simulink model "P702_NI_SoftECU"  (R2019a)
settings: Solver=ode1  StartTime=0.0  StopTime=Inf  FixedStep=0.001  RelTol=1e-3  EnableMultiTasking=on
PreLoadFcn:
  | run '.\VeriStand_BlockSet\NIVeriStandAddPaths.m'
undefined symbols (not defined in the file or in its folder): magnitude
libraries: simulink x83, simulink_extras x1
(part 68 of 76)

== system P702_NI_SoftECU/Output/Subsystem2/CAN_Signal/ECM_DIESEL PCM PCM_HEV/PowertrainData_1_0x421 ==
  AirCondFluidHi_P_Actl : Constant  Value=0
  CoolantFanStepAct : Constant  Value=0
  ECMMILRequest : Constant  Value=0
  EngIdlShutDown_D_Stat : Constant  Value=0
  EngIdlShutDwnTxt_D_Rq : Constant  Value=0
  FUEL_ALCOHOL_PERCNT : Constant  Value=0
  FohEng_D_Rq : Constant  Value=0
  OilPressureWarning : Constant  Value=0
  TrnTotLss_Tq_Est : Constant  Value=0
  TrnTotTq_Rt_Est : Constant  Value=0
  VehVLimActv_B_Actl : Constant  Value=0
  VehVLimStat_D_Actl : Constant  Value=0
  bus_creator : BusCreator  Inputs=12
  out_port : Outport
  wires:
  bus_creator/1 -> out_port/1  "Subsystem2"
  VehVLimActv_B_Actl/1 -> bus_creator/1  "VehVLimActv_B_Actl"
  VehVLimStat_D_Actl/1 -> bus_creator/2  "VehVLimStat_D_Actl"
  ECMMILRequest/1 -> bus_creator/3  "ECMMILRequest"
  FohEng_D_Rq/1 -> bus_creator/4  "FohEng_D_Rq"
  EngIdlShutDown_D_Stat/1 -> bus_creator/5  "EngIdlShutDown_D_Stat"
  CoolantFanStepAct/1 -> bus_creator/6  "CoolantFanStepAct"
  OilPressureWarning/1 -> bus_creator/7  "OilPressureWarning"
  EngIdlShutDwnTxt_D_Rq/1 -> bus_creator/8  "EngIdlShutDwnTxt_D_Rq"
  TrnTotLss_Tq_Est/1 -> bus_creator/9  "TrnTotLss_Tq_Est"
  TrnTotTq_Rt_Est/1 -> bus_creator/10  "TrnTotTq_Rt_Est"
  AirCondFluidHi_P_Actl/1 -> bus_creator/11  "AirCondFluidHi_P_Actl"
  FUEL_ALCOHOL_PERCNT/1 -> bus_creator/12  "FUEL_ALCOHOL_PERCNT"

== system P702_NI_SoftECU/Output/Subsystem2/CAN_Signal/ECM_DIESEL PCM PCM_HEV/PowertrainData_2_0x42D ==
  ApedPos_Pc_ActlDiag : Constant  Value=0
  EngAirIn_Te_Actl : Constant  Value=0
  EngClnt_Te_ActlDiag : Constant  Value=0
  EngLoad_Pc_CalcDiag : Constant  Value=0
  EngMsgTxt_D_Rq : Constant  Value=0
  GrllShtrPos_B_Falt : Constant  Value=0
  GrllShtrPos_D_Cmd : Constant  Value=0
  IsaOffst_D_Stat : Constant  Value=0
  ObdWarmUp_B_Complt : Constant  Value=0
  SlMde_D_RqDsply : Constant  Value=0
  SlMde_D_Stat : Constant  Value=0
  bus_creator : BusCreator  Inputs=11
  out_port : Outport
  wires:
  bus_creator/1 -> out_port/1  "Subsystem2"
  ObdWarmUp_B_Complt/1 -> bus_creator/1  "ObdWarmUp_B_Complt"
  EngMsgTxt_D_Rq/1 -> bus_creator/2  "EngMsgTxt_D_Rq"
  EngAirIn_Te_Actl/1 -> bus_creator/3  "EngAirIn_Te_Actl"
  ApedPos_Pc_ActlDiag/1 -> bus_creator/4  "ApedPos_Pc_ActlDiag"
  EngClnt_Te_ActlDiag/1 -> bus_creator/5  "EngClnt_Te_ActlDiag"
  EngLoad_Pc_CalcDiag/1 -> bus_creator/6  "EngLoad_Pc_CalcDiag"
  GrllShtrPos_D_Cmd/1 -> bus_creator/7  "GrllShtrPos_D_Cmd"
  GrllShtrPos_B_Falt/1 -> bus_creator/8  "GrllShtrPos_B_Falt"
  IsaOffst_D_Stat/1 -> bus_creator/9  "IsaOffst_D_Stat"
  SlMde_D_RqDsply/1 -> bus_creator/10  "SlMde_D_RqDsply"
  SlMde_D_Stat/1 -> bus_creator/11  "SlMde_D_Stat"

== system P702_NI_SoftECU/Output/Subsystem2/CAN_Signal/ECM_DIESEL PCM PCM_HEV/PowertrainData_3_0x43E ==
  BattULoChrg_U_Cmd : Constant  Value=0
  ElLoadCtl_D_Rq : Constant  Value=0
  EngMnfld_P_Actl : Constant  Value=0
  FuelPumpPwr_B_Rq : Constant  Value=0
  bus_creator : BusCreator  Inputs=4
  out_port : Outport
  wires:
  bus_creator/1 -> out_port/1  "Subsystem2"
  BattULoChrg_U_Cmd/1 -> bus_creator/1  "BattULoChrg_U_Cmd"
  ElLoadCtl_D_Rq/1 -> bus_creator/2  "ElLoadCtl_D_Rq"
  FuelPumpPwr_B_Rq/1 -> bus_creator/3  "FuelPumpPwr_B_Rq"
  EngMnfld_P_Actl/1 -> bus_creator/4  "EngMnfld_P_Actl"

== system P702_NI_SoftECU/Output/Subsystem2/CAN_Signal/ECM_DIESEL PCM PCM_HEV/PowertrainData_6_0x205 ==
  BrkTot_Tq_RqFapLc : Constant  Value=0
  FapLc_B_Err : Constant  Value=0
  TrnAin_Pc_RqDrv : Constant  Value=0
  bus_creator : BusCreator  Inputs=3
  out_port : Outport
  wires:
  bus_creator/1 -> out_port/1  "Subsystem2"
  BrkTot_Tq_RqFapLc/1 -> bus_creator/1  "BrkTot_Tq_RqFapLc"
  FapLc_B_Err/1 -> bus_creator/2  "FapLc_B_Err"
  TrnAin_Pc_RqDrv/1 -> bus_creator/3  "TrnAin_Pc_RqDrv"

== system P702_NI_SoftECU/Output/Subsystem2/CAN_Signal/ECM_DIESEL PCM PCM_HEV/PowertrainData_7_0x41F ==
  EcoCochA_Pc_Dsply : Constant  Value=0
  EcoCochCrus_Pc_Dsply : Constant  Value=0
  EcoCochDecel_Pc_Dsply : Constant  Value=0
  EcoCochIdlFuel_Pc_Dsply : Constant  Value=0
  EcoCochInstNeg_B_Dsply : Constant  Value=0
  EcoCochInst_Pc_Dsply : Constant  Value=0
  EcoCochShif_Pc_Dsply : Constant  Value=0
  bus_creator : BusCreator  Inputs=7
  out_port : Outport
  wires:
  bus_creator/1 -> out_port/1  "Subsystem2"
  EcoCochA_Pc_Dsply/1 -> bus_creator/1  "EcoCochA_Pc_Dsply"
  EcoCochCrus_Pc_Dsply/1 -> bus_creator/2  "EcoCochCrus_Pc_Dsply"
  EcoCochDecel_Pc_Dsply/1 -> bus_creator/3  "EcoCochDecel_Pc_Dsply"
  EcoCochIdlFuel_Pc_Dsply/1 -> bus_creator/4  "EcoCochIdlFuel_Pc_Dsply"
  EcoCochShif_Pc_Dsply/1 -> bus_creator/5  "EcoCochShif_Pc_Dsply"
  EcoCochInst_Pc_Dsply/1 -> bus_creator/6  "EcoCochInst_Pc_Dsply"
  EcoCochInstNeg_B_Dsply/1 -> bus_creator/7  "EcoCochInstNeg_B_Dsply"

== system P702_NI_SoftECU/Output/Subsystem2/CAN_Signal/ECM_DIESEL PCM PCM_HEV/PowertrainData_9_0x44C ==
  AutoTowActv_B_Stat : Constant  Value=0
  AutoTowAllw_D_StatMnu : Constant  Value=0
  GrossTrainWeight_M_Est : Constant  Value=0
  TrailCtlPt_B_Falt : Constant  Value=0
  Veh_V_DsplyTrailCtlSet : Constant  Value=0
  WakeAlarm1_B_Typ : Constant  Value=0
  WakeAlarm1_T_Rq : Constant  Value=0
  bus_creator : BusCreator  Inputs=7
  out_port : Outport
  wires:
  bus_creator/1 -> out_port/1  "Subsystem2"
  GrossTrainWeight_M_Est/1 -> bus_creator/1  "GrossTrainWeight_M_Est"
  AutoTowAllw_D_StatMnu/1 -> bus_creator/2  "AutoTowAllw_D_StatMnu"
  AutoTowActv_B_Stat/1 -> bus_creator/3  "AutoTowActv_B_Stat"
  TrailCtlPt_B_Falt/1 -> bus_creator/4  "TrailCtlPt_B_Falt"
  Veh_V_DsplyTrailCtlSet/1 -> bus_creator/5  "Veh_V_DsplyTrailCtlSet"
  WakeAlarm1_T_Rq/1 -> bus_creator/6  "WakeAlarm1_T_Rq"
  WakeAlarm1_B_Typ/1 -> bus_creator/7  "WakeAlarm1_B_Typ"

== system P702_NI_SoftECU/Output/Subsystem2/CAN_Signal/ECM_DIESEL PCM PCM_HEV/Powertrain_Data_4_0x424 ==
  BpedDrvMsgTxt_B_Dsply : Constant  Value=0
  FuelLvlWarn_D_ActlEng : Constant  Value=0
  FuelLvl_Pc_DsplyEng : Constant  Value=0
  FuelRange_L_DsplyEng : Constant  Value=0
  RearDiffOilTeWarn_B_Rq : Constant  Value=0
  RearDiffOil_Te_Actl : Constant  Value=0
  SelDrvMdePt_D_Stat : Constant  Value=0
  bus_creator : BusCreator  Inputs=7
  out_port : Outport
  wires:
  bus_creator/1 -> out_port/1  "Subsystem2"
  BpedDrvMsgTxt_B_Dsply/1 -> bus_creator/1  "BpedDrvMsgTxt_B_Dsply"
  RearDiffOil_Te_Actl/1 -> bus_creator/2  "RearDiffOil_Te_Actl"
  RearDiffOilTeWarn_B_Rq/1 -> bus_creator/3  "RearDiffOilTeWarn_B_Rq"
  FuelLvlWarn_D_ActlEng/1 -> bus_creator/4  "FuelLvlWarn_D_ActlEng"
  SelDrvMdePt_D_Stat/1 -> bus_creator/5  "SelDrvMdePt_D_Stat"
  FuelRange_L_DsplyEng/1 -> bus_creator/6  "FuelRange_L_DsplyEng"
  FuelLvl_Pc_DsplyEng/1 -> bus_creator/7  "FuelLvl_Pc_DsplyEng"

== system P702_NI_SoftECU/Output/Subsystem2/CAN_Signal/ECM_DIESEL PCM PCM_HEV/Powertrain_Data_5_0x43F ==
  FapLcActv_B_Stat : Constant  Value=0
  FapLcInhbt_B_Rq : Constant  Value=0
  FapLcMaxGrdAbrt_B_Stat : Constant  Value=0
  FapLcMaxGrdInhbt_B_Stat : Constant  Value=0
  FapLcObstcl_B_Stat : Constant  Value=0
  FapLcPrchgBrk_B_Rq : Constant  Value=0
  FapLcStopHold_B_Rq : Constant  Value=0
  bus_creator : BusCreator  Inputs=7
  out_port : Outport
  wires:
  bus_creator/1 -> out_port/1  "Subsystem2"
  FapLcActv_B_Stat/1 -> bus_creator/1  "FapLcActv_B_Stat"
  FapLcMaxGrdAbrt_B_Stat/1 -> bus_creator/2  "FapLcMaxGrdAbrt_B_Stat"
  FapLcMaxGrdInhbt_B_Stat/1 -> bus_creator/3  "FapLcMaxGrdInhbt_B_Stat"
  FapLcObstcl_B_Stat/1 -> bus_creator/4  "FapLcObstcl_B_Stat"
  FapLcPrchgBrk_B_Rq/1 -> bus_creator/5  "FapLcPrchgBrk_B_Rq"
  FapLcStopHold_B_Rq/1 -> bus_creator/6  "FapLcStopHold_B_Rq"
  FapLcInhbt_B_Rq/1 -> bus_creator/7  "FapLcInhbt_B_Rq"

== system P702_NI_SoftECU/Output/Subsystem2/CAN_Signal/ECM_DIESEL PCM PCM_HEV/Stop_Start_0x166 ==
  AutoStopPtDelta_I_Est : Constant  Value=0
  HiElPwInhbt_B_Stat : Constant  Value=0
  OdoTripVerify_L_Actl : Constant  Value=0
  StopStrtDrvMde_D_Indic : Constant  Value=0
  StopStrtIODTxt_D_Rq : Constant  Value=0
  StopStrtMsgTxt_D_Rq : Constant  Value=0
  StopStrtStdby_D_Indic : Constant  Value=0
  bus_creator : BusCreator  Inputs=7
  out_port : Outport
  wires:
  bus_creator/1 -> out_port/1  "Subsystem2"
  AutoStopPtDelta_I_Est/1 -> bus_creator/1  "AutoStopPtDelta_I_Est"
  HiElPwInhbt_B_Stat/1 -> bus_creator/2  "HiElPwInhbt_B_Stat"
  StopStrtDrvMde_D_Indic/1 -> bus_creator/3  "StopStrtDrvMde_D_Indic"
  StopStrtMsgTxt_D_Rq/1 -> bus_creator/4  "StopStrtMsgTxt_D_Rq"
  OdoTripVerify_L_Actl/1 -> bus_creator/5  "OdoTripVerify_L_Actl"
  StopStrtStdby_D_Indic/1 -> bus_creator/6  "StopStrtStdby_D_Indic"
  StopStrtIODTxt_D_Rq/1 -> bus_creator/7  "StopStrtIODTxt_D_Rq"

== system P702_NI_SoftECU/Output/Subsystem2/CAN_Signal/ECM_DIESEL PCM PCM_HEV/TesterPhysicalResPCM_0x7E8 ==
  TesterPhysicalResPCM : Constant  Value=0
  bus_creator : BusCreator  Inputs=1
  out_port : Outport
  wires:
  bus_creator/1 -> out_port/1  "Subsystem2"
  TesterPhysicalResPCM/1 -> bus_creator/1  "TesterPhysicalResPCM"

== system P702_NI_SoftECU/Output/Subsystem2/CAN_Signal/ECM_DIESEL PCM PCM_HEV/TorqueDataEngFlags_0x200 ==
  PrplWhlTotTqRq_No_Cnt : Constant  Value=0
  PrplWhlTotTqRq_No_Cs : Constant  Value=0
  PrplWhlTot_Tq_LimMn : Constant  Value=0
  PrplWhlTot_Tq_Rq : Constant  Value=0
  PtDrvMde_D_Stat : Constant  Value=0
  bus_creator : BusCreator  Inputs=5
  out_port : Outport
  wires:
  bus_creator/1 -> out_port/1  "Subsystem2"
  PrplWhlTot_Tq_LimMn/1 -> bus_creator/1  "PrplWhlTot_Tq_LimMn"
  PrplWhlTot_Tq_Rq/1 -> bus_creator/2  "PrplWhlTot_Tq_Rq"
  PtDrvMde_D_Stat/1 -> bus_creator/3  "PtDrvMde_D_Stat"
  PrplWhlTotTqRq_No_Cnt/1 -> bus_creator/4  "PrplWhlTotTqRq_No_Cnt"
  PrplWhlTotTqRq_No_Cs/1 -> bus_creator/5  "PrplWhlTotTqRq_No_Cs"

== system P702_NI_SoftECU/Output/Subsystem2/CAN_Signal/ECM_DIESEL PCM PCM_HEV/TransGearData ==
  GboxOil_Te_Actl : Constant  Value=0
  GearLvrPos_D_Actl : Constant  Value=0
  SelDrvMdeSwtch_D_Stat3 : Constant  Value=0
  TrnShifActv_B_Actl : Constant  Value=0
  TrnSrvcRqd_B_Rq : Constant  Value=0
  bus_creator : BusCreator  Inputs=5
  out_port : Outport
  wires:
  bus_creator/1 -> out_port/1  "Subsystem2"
  GboxOil_Te_Actl/1 -> bus_creator/1  "GboxOil_Te_Actl"
  GearLvrPos_D_Actl/1 -> bus_creator/2  "GearLvrPos_D_Actl"
  SelDrvMdeSwtch_D_Stat3/1 -> bus_creator/3  "SelDrvMdeSwtch_D_Stat3"
  TrnShifActv_B_Actl/1 -> bus_creator/4  "TrnShifActv_B_Actl"
  TrnSrvcRqd_B_Rq/1 -> bus_creator/5  "TrnSrvcRqd_B_Rq"

== system P702_NI_SoftECU/Output/Subsystem2/CAN_Signal/ECM_DIESEL PCM PCM_HEV/VehicleOperatingModes_0x167 ==
  ElPw_D_Stat : Constant  Value=0
  ElPw_D_StatStrtStop : Constant  Value=0
  Eng_D_Stat : Constant  Value=0
  PlgActvArb_B_Actl : Constant  Value=0
  PrplWhlRgenMn_Tq_Actl : Constant  Value=0
  PrplWhlTot2_Tq_Actl : Constant  Value=0
  PwPckTq_D_Stat : Constant  Value=0
  TrnAinTq_D_Qf : Constant  Value=0
  TrnAin_Tq_Actl : Constant  Value=0
  bus_creator : BusCreator  Inputs=9
  out_port : Outport
  wires:
  bus_creator/1 -> out_port/1  "Subsystem2"
  Eng_D_Stat/1 -> bus_creator/1  "Eng_D_Stat"
  PwPckTq_D_Stat/1 -> bus_creator/2  "PwPckTq_D_Stat"
  ElPw_D_Stat/1 -> bus_creator/3  "ElPw_D_Stat"
  PlgActvArb_B_Actl/1 -> bus_creator/4  "PlgActvArb_B_Actl"
  PrplWhlTot2_Tq_Actl/1 -> bus_creator/5  "PrplWhlTot2_Tq_Actl"
  ElPw_D_StatStrtStop/1 -> bus_creator/6  "ElPw_D_StatStrtStop"
  PrplWhlRgenMn_Tq_Actl/1 -> bus_creator/7  "PrplWhlRgenMn_Tq_Actl"
  TrnAinTq_D_Qf/1 -> bus_creator/8  "TrnAinTq_D_Qf"
  TrnAin_Tq_Actl/1 -> bus_creator/9  "TrnAin_Tq_Actl"

== system P702_NI_SoftECU/Output/Subsystem2/CAN_Signal/GWM/GSM ==
  in : Inport
  Gear_Shift_by_Wire_2_FD1_168 : Subsystem
  Gear_Shift_by_Wire_FD1_5A : Subsystem
  bus_creator : BusCreator  Inputs=2
  bus_selector : BusSelector  OutputSignals=Gear_Shift_by_Wire_2_FD1_168,Gear_Shift_by_Wire_FD1_5A
  out_port : Outport
  wires:
  bus_creator/1 -> out_port/1  "Subsystem2"
  Gear_Shift_by_Wire_2_FD1_168/1(out_port) -> bus_creator/1  "Gear_Shift_by_Wire_2_FD1_168"
  Gear_Shift_by_Wire_FD1_5A/1(out_port) -> bus_creator/2  "Gear_Shift_by_Wire_FD1_5A"
  in/1 -> bus_selector/1

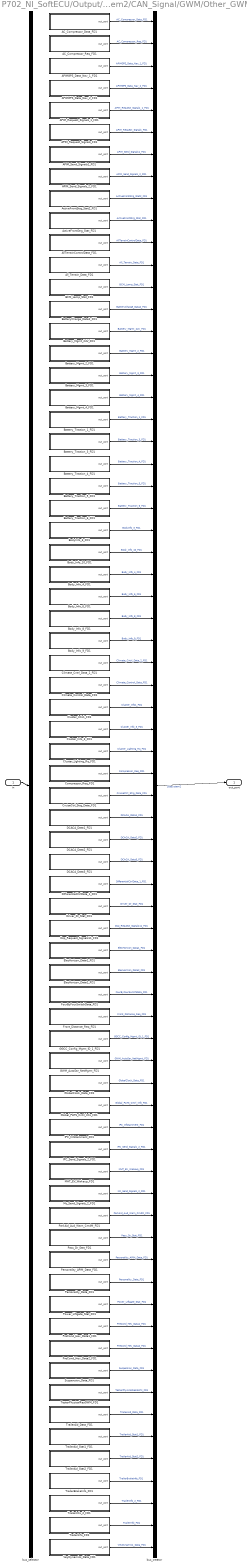
== system P702_NI_SoftECU/Output/Subsystem2/CAN_Signal/GWM/Other_GWMTx ==
  in : Inport
  AC_Compressor_Data_FD1 : Subsystem
  AC_Compressor_Req_FD1 : Subsystem
  APIMGPS_Data_Nav_1_FD1 : Subsystem
  APIMGPS_Data_Nav_2_FD1 : Subsystem
  APIM_Request_Signals_1_FD1 : Subsystem
  APIM_Request_Signals_FD1 : Subsystem
  APIM_Send_Signals1_FD1 : Subsystem
  APIM_Send_Signals_2_FD1 : Subsystem
  ActiveFrontStrg_Stat2_FD1 : Subsystem
  ActiveFrontStrg_Stat_FD1 : Subsystem
  AllTerrainControlData_FD1 : Subsystem
  All_Terrain_Data_FD1 : Subsystem
  BCM_Lamp_Stat_FD1 : Subsystem
  BatteryCharge_Data2_FD1 : Subsystem
  Battery_Mgmt_24V_FD1 : Subsystem
  Battery_Mgmt_2_FD1 : Subsystem
  Battery_Mgmt_3_FD1 : Subsystem
  Battery_Mgmt_4_FD1 : Subsystem
  Battery_Traction_1_FD1 : Subsystem
  Battery_Traction_3_FD1 : Subsystem
  Battery_Traction_4_FD1 : Subsystem
  Battery_Traction_5_FD1 : Subsystem
  Battery_Traction_6_FD1 : Subsystem
  BodyInfo_3_FD1 : Subsystem
  Body_Info_10_FD1 : Subsystem
  Body_Info_4_FD1 : Subsystem
  Body_Info_6_FD1 : Subsystem
  Body_Info_8_FD1 : Subsystem
  Body_Info_9_FD1 : Subsystem
  Climate_Cntrl_Data_2_FD1 : Subsystem
  Climate_Control_Data_FD1 : Subsystem
  Cluster_Info1_FD1 : Subsystem
  Cluster_Info_3_FD1 : Subsystem
  Cluster_Lighting_Rq_FD1 : Subsystem
  Compressor_Req_FD1 : Subsystem
  CruiseCtrl_Strg_Data_FD1 : Subsystem
  DCACA_Data1_FD1 : Subsystem
  DCACA_Data2_FD1 : Subsystem
  DCACA_Data3_FD1 : Subsystem
  DifferentialCtrlData_1_FD1 : Subsystem
  Driver_Dr_Stat_FD1 : Subsystem
  Dsp_Request_Signals11_FD1 : Subsystem
  ElecHorizon_Data1_FD1 : Subsystem
  ElecHorizon_Data2_FD1 : Subsystem
  FourByFourSwitchData_FD1 : Subsystem
  Front_Distance_Req_FD1 : Subsystem
  GGCC_Config_Mgmt_ID_1_FD1 : Subsystem
  GWM_AutoSar_NetMgmt_FD1 : Subsystem
  GlobalClock_Data_FD1 : Subsystem
  Global_PATS_Cntrl_Info_FD1 : Subsystem
  IPC_Infotainment_FD1 : Subsystem
  IPC_Send_Signals_2_FD1 : Subsystem
  MHT_EV_Wakeup_FD1 : Subsystem
  Mc_Send_Signals_2_FD1 : Subsystem
  ParkAid_Aud_Warn_CmdM_FD1 : Subsystem
  Pass_Dr_Stat_FD1 : Subsystem
  Personality_APIM_Data_FD1 : Subsystem
  Personality_Data_FD1 : Subsystem
  Power_Liftgate_Stat_FD1 : Subsystem
  PreCond_Hev_Data1_FD1 : Subsystem
  PreCond_Hev_Data2_FD1 : Subsystem
  Suspension_Data_FD1 : Subsystem
  TesterPhysicalResGWM_FD1 : Subsystem
  TrailerAid_Data_FD1 : Subsystem
  TrailerAid_Stat1_FD1 : Subsystem
  TrailerAid_Stat2_FD1 : Subsystem
  TrailerBrakeInfo_FD1 : Subsystem
  TrailerInfo_2_FD1 : Subsystem
  TrailerInfo_FD1 : Subsystem
  VeyDynamics_Data_FD1 : Subsystem
  bus_creator : BusCreator  Inputs=70
  bus_selector : BusSelector  OutputSignals=AC_Compressor_Data_FD1,AC_Compressor_Req_FD1,APIMGPS_Data_Nav_1_FD1,APIMGPS_Data_Nav_2_FD1,APIM_Request_Signals_1_FD1,APIM_Request_Signals_FD1,APIM_Send_Signals1_FD1,APIM_Send_Signals_2_FD1,ActiveFrontStrg_Stat2_FD1,ActiveFrontStrg_Stat_FD1,AllTerrainControlData_FD1,All_Terrain_Data_FD1,BCM_Lamp_Stat_FD1,BatteryCharge_Data2_FD1,Battery_Mgmt_24V_FD1,Battery_Mgmt_2_FD1,Battery_Mgmt_3_FD1,Battery_Mgmt_4_FD1,Battery_Traction_1_FD1,Battery_Traction_3_FD1,Battery_Traction_4_FD1,Battery_Traction_5_FD1,Battery_Traction_6_FD1,BodyInfo_3_FD1,Body_Info_10_FD1,Body_Info_4_FD1,Body_Info_6_FD1,Body_Info_8_FD1,Body_Info_9_FD1,Climate_Cntrl_Data_2_FD1,Climate_Control_Data_FD1,Cluster_Info1_FD1,Cluster_Info_3_FD1,Cluster_Lighting_Rq_FD1,Compressor_Req_FD1,CruiseCtrl_Strg_Data_FD1,DCACA_Data1_FD1,DCACA_Data2_FD1,DCACA_Data3_FD1,DifferentialCtrlData_1_FD1,Driver_Dr_Stat_FD1,Dsp_Request_Signals11_FD1,ElecHorizon_Data1_FD1,ElecHorizon_Data2_FD1,FourByFourSwitchData_FD1,Front_Distance_Req_FD1,GGCC_Config_Mgmt_ID_1_FD1,GWM_AutoSar_NetMgmt_FD1,GlobalClock_Data_FD1,Global_PATS_Cntrl_Info_FD1,IPC_Infotainment_FD1,IPC_Send_Signals_2_FD1,MHT_EV_Wakeup_FD1,Mc_Send_Signals_2_FD1,ParkAid_Aud_Warn_CmdM_FD1,Pass_Dr_Stat_FD1,Personality_APIM_Data_FD1,Personality_Data_FD1,Power_Liftgate_Stat_FD1,PreCond_Hev_Data1_FD1,PreCond_Hev_Data2_FD1,Suspension_Data_FD1,TesterPhysicalResGWM_FD1,TrailerAid_Data_FD1,TrailerAid_Stat1_FD1,TrailerAid_Stat2_FD1,TrailerBrakeInfo_FD1,TrailerInfo_2_FD1,TrailerInfo_FD1,VeyDynamics_Data_FD1
  out_port : Outport
  wires:
  bus_creator/1 -> out_port/1  "Subsystem2"
  AC_Compressor_Data_FD1/1(out_port) -> bus_creator/1  "AC_Compressor_Data_FD1"
  AC_Compressor_Req_FD1/1(out_port) -> bus_creator/2  "AC_Compressor_Req_FD1"
  APIMGPS_Data_Nav_1_FD1/1(out_port) -> bus_creator/3  "APIMGPS_Data_Nav_1_FD1"
  APIMGPS_Data_Nav_2_FD1/1(out_port) -> bus_creator/4  "APIMGPS_Data_Nav_2_FD1"
  APIM_Request_Signals_1_FD1/1(out_port) -> bus_creator/5  "APIM_Request_Signals_1_FD1"
  APIM_Request_Signals_FD1/1(out_port) -> bus_creator/6  "APIM_Request_Signals_FD1"
  APIM_Send_Signals1_FD1/1(out_port) -> bus_creator/7  "APIM_Send_Signals1_FD1"
  APIM_Send_Signals_2_FD1/1(out_port) -> bus_creator/8  "APIM_Send_Signals_2_FD1"
  ActiveFrontStrg_Stat2_FD1/1(out_port) -> bus_creator/9  "ActiveFrontStrg_Stat2_FD1"
  ActiveFrontStrg_Stat_FD1/1(out_port) -> bus_creator/10  "ActiveFrontStrg_Stat_FD1"
  AllTerrainControlData_FD1/1(out_port) -> bus_creator/11  "AllTerrainControlData_FD1"
  All_Terrain_Data_FD1/1(out_port) -> bus_creator/12  "All_Terrain_Data_FD1"
  BCM_Lamp_Stat_FD1/1(out_port) -> bus_creator/13  "BCM_Lamp_Stat_FD1"
  BatteryCharge_Data2_FD1/1(out_port) -> bus_creator/14  "BatteryCharge_Data2_FD1"
  Battery_Mgmt_24V_FD1/1(out_port) -> bus_creator/15  "Battery_Mgmt_24V_FD1"
  Battery_Mgmt_2_FD1/1(out_port) -> bus_creator/16  "Battery_Mgmt_2_FD1"
  Battery_Mgmt_3_FD1/1(out_port) -> bus_creator/17  "Battery_Mgmt_3_FD1"
  Battery_Mgmt_4_FD1/1(out_port) -> bus_creator/18  "Battery_Mgmt_4_FD1"
  Battery_Traction_1_FD1/1(out_port) -> bus_creator/19  "Battery_Traction_1_FD1"
  Battery_Traction_3_FD1/1(out_port) -> bus_creator/20  "Battery_Traction_3_FD1"
  Battery_Traction_4_FD1/1(out_port) -> bus_creator/21  "Battery_Traction_4_FD1"
  Battery_Traction_5_FD1/1(out_port) -> bus_creator/22  "Battery_Traction_5_FD1"
  Battery_Traction_6_FD1/1(out_port) -> bus_creator/23  "Battery_Traction_6_FD1"
  BodyInfo_3_FD1/1(out_port) -> bus_creator/24  "BodyInfo_3_FD1"
  Body_Info_10_FD1/1(out_port) -> bus_creator/25  "Body_Info_10_FD1"
  Body_Info_4_FD1/1(out_port) -> bus_creator/26  "Body_Info_4_FD1"
  Body_Info_6_FD1/1(out_port) -> bus_creator/27  "Body_Info_6_FD1"
  Body_Info_8_FD1/1(out_port) -> bus_creator/28  "Body_Info_8_FD1"
  Body_Info_9_FD1/1(out_port) -> bus_creator/29  "Body_Info_9_FD1"
  Climate_Cntrl_Data_2_FD1/1(out_port) -> bus_creator/30  "Climate_Cntrl_Data_2_FD1"
  Climate_Control_Data_FD1/1(out_port) -> bus_creator/31  "Climate_Control_Data_FD1"
  Cluster_Info1_FD1/1(out_port) -> bus_creator/32  "Cluster_Info1_FD1"
  Cluster_Info_3_FD1/1(out_port) -> bus_creator/33  "Cluster_Info_3_FD1"
  Cluster_Lighting_Rq_FD1/1(out_port) -> bus_creator/34  "Cluster_Lighting_Rq_FD1"
  Compressor_Req_FD1/1(out_port) -> bus_creator/35  "Compressor_Req_FD1"
  CruiseCtrl_Strg_Data_FD1/1(out_port) -> bus_creator/36  "CruiseCtrl_Strg_Data_FD1"
  DCACA_Data1_FD1/1(out_port) -> bus_creator/37  "DCACA_Data1_FD1"
  DCACA_Data2_FD1/1(out_port) -> bus_creator/38  "DCACA_Data2_FD1"
  DCACA_Data3_FD1/1(out_port) -> bus_creator/39  "DCACA_Data3_FD1"
  DifferentialCtrlData_1_FD1/1(out_port) -> bus_creator/40  "DifferentialCtrlData_1_FD1"
  Driver_Dr_Stat_FD1/1(out_port) -> bus_creator/41  "Driver_Dr_Stat_FD1"
  Dsp_Request_Signals11_FD1/1(out_port) -> bus_creator/42  "Dsp_Request_Signals11_FD1"
  ElecHorizon_Data1_FD1/1(out_port) -> bus_creator/43  "ElecHorizon_Data1_FD1"
  ElecHorizon_Data2_FD1/1(out_port) -> bus_creator/44  "ElecHorizon_Data2_FD1"
  FourByFourSwitchData_FD1/1(out_port) -> bus_creator/45  "FourByFourSwitchData_FD1"
  Front_Distance_Req_FD1/1(out_port) -> bus_creator/46  "Front_Distance_Req_FD1"
  GGCC_Config_Mgmt_ID_1_FD1/1(out_port) -> bus_creator/47  "GGCC_Config_Mgmt_ID_1_FD1"
  GWM_AutoSar_NetMgmt_FD1/1(out_port) -> bus_creator/48  "GWM_AutoSar_NetMgmt_FD1"
  GlobalClock_Data_FD1/1(out_port) -> bus_creator/49  "GlobalClock_Data_FD1"
  Global_PATS_Cntrl_Info_FD1/1(out_port) -> bus_creator/50  "Global_PATS_Cntrl_Info_FD1"
  IPC_Infotainment_FD1/1(out_port) -> bus_creator/51  "IPC_Infotainment_FD1"
  IPC_Send_Signals_2_FD1/1(out_port) -> bus_creator/52  "IPC_Send_Signals_2_FD1"
  MHT_EV_Wakeup_FD1/1(out_port) -> bus_creator/53  "MHT_EV_Wakeup_FD1"
  Mc_Send_Signals_2_FD1/1(out_port) -> bus_creator/54  "Mc_Send_Signals_2_FD1"
  ParkAid_Aud_Warn_CmdM_FD1/1(out_port) -> bus_creator/55  "ParkAid_Aud_Warn_CmdM_FD1"
  Pass_Dr_Stat_FD1/1(out_port) -> bus_creator/56  "Pass_Dr_Stat_FD1"
  Personality_APIM_Data_FD1/1(out_port) -> bus_creator/57  "Personality_APIM_Data_FD1"
  Personality_Data_FD1/1(out_port) -> bus_creator/58  "Personality_Data_FD1"
  Power_Liftgate_Stat_FD1/1(out_port) -> bus_creator/59  "Power_Liftgate_Stat_FD1"
  PreCond_Hev_Data1_FD1/1(out_port) -> bus_creator/60  "PreCond_Hev_Data1_FD1"
  PreCond_Hev_Data2_FD1/1(out_port) -> bus_creator/61  "PreCond_Hev_Data2_FD1"
  Suspension_Data_FD1/1(out_port) -> bus_creator/62  "Suspension_Data_FD1"
  TesterPhysicalResGWM_FD1/1(out_port) -> bus_creator/63  "TesterPhysicalResGWM_FD1"
  TrailerAid_Data_FD1/1(out_port) -> bus_creator/64  "TrailerAid_Data_FD1"
  TrailerAid_Stat1_FD1/1(out_port) -> bus_creator/65  "TrailerAid_Stat1_FD1"
  TrailerAid_Stat2_FD1/1(out_port) -> bus_creator/66  "TrailerAid_Stat2_FD1"
  TrailerBrakeInfo_FD1/1(out_port) -> bus_creator/67  "TrailerBrakeInfo_FD1"
  TrailerInfo_2_FD1/1(out_port) -> bus_creator/68  "TrailerInfo_2_FD1"
  TrailerInfo_FD1/1(out_port) -> bus_creator/69  "TrailerInfo_FD1"
  VeyDynamics_Data_FD1/1(out_port) -> bus_creator/70  "VeyDynamics_Data_FD1"
  in/1 -> bus_selector/1

== system P702_NI_SoftECU/Output/Subsystem2/CAN_Signal/GWM/RCM ==
  in : Inport
  RCMSerialNumber_FD1_454 : Subsystem
  RCMStatusMessage2_FD1_4C : Subsystem
  bus_creator : BusCreator  Inputs=2
  bus_selector : BusSelector  OutputSignals=RCMStatusMessage2_FD1_4C,RCMSerialNumber_FD1_454
  out_port : Outport
  wires:
  bus_creator/1 -> out_port/1  "Subsystem2"
  RCMStatusMessage2_FD1_4C/1(out_port) -> bus_creator/1  "RCMStatusMessage2_FD1_4C"
  RCMSerialNumber_FD1_454/1(out_port) -> bus_creator/2  "RCMSerialNumber_FD1_454"
  in/1 -> bus_selector/1

== system P702_NI_SoftECU/Output/Subsystem2/CAN_Signal/GWM/SCCM ==
  in : Inport
  Steering_Data_FD1_83 : Subsystem
  Steering_Wheel_Data2_FD1_81 : Subsystem
  bus_creator : BusCreator  Inputs=2
  bus_selector : BusSelector  OutputSignals=Steering_Data_FD1_83,Steering_Wheel_Data2_FD1_81
  out_port : Outport
  wires:
  bus_creator/1 -> out_port/1  "Subsystem2"
  Steering_Data_FD1_83/1(out_port) -> bus_creator/1  "Steering_Data_FD1_83"
  Steering_Wheel_Data2_FD1_81/1(out_port) -> bus_creator/2  "Steering_Wheel_Data2_FD1_81"
  in/1 -> bus_selector/1

== system P702_NI_SoftECU/Output/Subsystem2/CAN_Signal/GWM/Tester//AutoSar ==
  in : Inport
  GWM_AutoSar_NetMgmt_FD1 : Subsystem
  TesterPhysicalResGWM_FD1 : Subsystem
  bus_creator : BusCreator  Inputs=2
  bus_selector : BusSelector  OutputSignals=GWM_AutoSar_NetMgmt_FD1,TesterPhysicalResGWM_FD1
  out_port : Outport
  wires:
  bus_creator/1 -> out_port/1  "Subsystem2"
  GWM_AutoSar_NetMgmt_FD1/1(out_port) -> bus_creator/1  "GWM_AutoSar_NetMgmt_FD1"
  TesterPhysicalResGWM_FD1/1(out_port) -> bus_creator/2  "TesterPhysicalResGWM_FD1"
  in/1 -> bus_selector/1

== system P702_NI_SoftECU/Output/Subsystem2/CAN_Signal/PSCM/EPAS_INFO_0x82 ==
  DrvSteActv_B_Stat : Constant  Value=0
  DrvSte_Tq_Actl : Constant  Value=0
  EPAS_Failure : Constant  Value=0
  SAPPAngleControlStat{1..6} (6 alike) : Constant  Value=0
  SteMdule_D_Stat : Constant  Value=0
  SteMdule_I_Est : Constant  Value=0
  SteMdule_U_Meas : Constant  Value=0
  SteeringColumnTorque : Constant  Value=0
  TrlrHitchLamp_D_Rqst : Constant  Value=0
  VehVTrlrAid_B_Rq : Constant  Value=0
  Veh_V_RqMxTrlrAid : Constant  Value=0
  bus_creator : BusCreator  Inputs=16
  out_port : Outport
  wires:
  bus_creator/1 -> out_port/1  "Subsystem2"
  SteeringColumnTorque/1 -> bus_creator/1  "SteeringColumnTorque"
  SAPPAngleControlStat6/1 -> bus_creator/2  "SAPPAngleControlStat6"
  SAPPAngleControlStat5/1 -> bus_creator/3  "SAPPAngleControlStat5"
  SAPPAngleControlStat4/1 -> bus_creator/4  "SAPPAngleControlStat4"
  SAPPAngleControlStat3/1 -> bus_creator/5  "SAPPAngleControlStat3"
  SAPPAngleControlStat2/1 -> bus_creator/6  "SAPPAngleControlStat2"
  DrvSteActv_B_Stat/1 -> bus_creator/7  "DrvSteActv_B_Stat"
  EPAS_Failure/1 -> bus_creator/8  "EPAS_Failure"
  SAPPAngleControlStat1/1 -> bus_creator/9  "SAPPAngleControlStat1"
  SteMdule_I_Est/1 -> bus_creator/10  "SteMdule_I_Est"
  VehVTrlrAid_B_Rq/1 -> bus_creator/11  "VehVTrlrAid_B_Rq"
  TrlrHitchLamp_D_Rqst/1 -> bus_creator/12  "TrlrHitchLamp_D_Rqst"
  SteMdule_U_Meas/1 -> bus_creator/13  "SteMdule_U_Meas"
  DrvSte_Tq_Actl/1 -> bus_creator/14  "DrvSte_Tq_Actl"
  SteMdule_D_Stat/1 -> bus_creator/15  "SteMdule_D_Stat"
  Veh_V_RqMxTrlrAid/1 -> bus_creator/16  "Veh_V_RqMxTrlrAid"

== system P702_NI_SoftECU/Output/Subsystem2/CAN_Signal/PSCM/Lane_Assist_Data3_FD1_0x3CC ==
  LaActAvail_D_Actl : Constant  Value=0
  LaActDeny_B_Actl : Constant  Value=0
  LaHandsOff_B_Actl : Constant  Value=0
  LsmcBrkDecelEnbl_D_Rq : Constant  Value=0
  LsmcBrk_Tq_Rq : Constant  Value=0
  TjaHandsOnCnfdnc_B_Est : Constant  Value=0
  TrlrAn_An_TrgtCalc : Constant  Value=0
  bus_creator : BusCreator  Inputs=7
  out_port : Outport
  wires:
  bus_creator/1 -> out_port/1  "Subsystem2"
  LaHandsOff_B_Actl/1 -> bus_creator/1  "LaHandsOff_B_Actl"
  LaActDeny_B_Actl/1 -> bus_creator/2  "LaActDeny_B_Actl"
  LaActAvail_D_Actl/1 -> bus_creator/3  "LaActAvail_D_Actl"
  TjaHandsOnCnfdnc_B_Est/1 -> bus_creator/4  "TjaHandsOnCnfdnc_B_Est"
  LsmcBrkDecelEnbl_D_Rq/1 -> bus_creator/5  "LsmcBrkDecelEnbl_D_Rq"
  LsmcBrk_Tq_Rq/1 -> bus_creator/6  "LsmcBrk_Tq_Rq"
  TrlrAn_An_TrgtCalc/1 -> bus_creator/7  "TrlrAn_An_TrgtCalc"

== system P702_NI_SoftECU/Output/Subsystem2/CAN_Signal/PSCM/PSCM_AutoSar_NetwrkMgmt_0x5B5 ==
  PSCM_AutoSarNMControl : Constant  Value=0
  PSCM_AutoSarNMNodeId : Constant  Value=0
  PSCM_AutoSarNMReserved{1..4} (4 alike) : Constant  Value=0
  PSCM_GWNMProxy : Constant  Value=0
  PSCM_GWOnBoardTester : Constant  Value=0
  bus_creator : BusCreator  Inputs=8
  out_port : Outport
  wires:
  bus_creator/1 -> out_port/1  "Subsystem2"
  PSCM_AutoSarNMNodeId/1 -> bus_creator/1  "PSCM_AutoSarNMNodeId"
  PSCM_AutoSarNMControl/1 -> bus_creator/2  "PSCM_AutoSarNMControl"
  PSCM_AutoSarNMReserved1/1 -> bus_creator/3  "PSCM_AutoSarNMReserved1"
  PSCM_AutoSarNMReserved2/1 -> bus_creator/4  "PSCM_AutoSarNMReserved2"
  PSCM_GWOnBoardTester/1 -> bus_creator/5  "PSCM_GWOnBoardTester"
  PSCM_GWNMProxy/1 -> bus_creator/6  "PSCM_GWNMProxy"
  PSCM_AutoSarNMReserved3/1 -> bus_creator/7  "PSCM_AutoSarNMReserved3"
  PSCM_AutoSarNMReserved4/1 -> bus_creator/8  "PSCM_AutoSarNMReserved4"

== system P702_NI_SoftECU/Output/Subsystem2/CAN_Signal/PSCM/SteeringPinion_Data_0x7E ==
  StePinAn_No_Cnt : Constant  Value=0
  StePinAn_No_Cs : Constant  Value=0
  StePinCompAnEst_D_Qf : Constant  Value=0
  StePinComp_An_Est : Constant  Value=0
  StePinRelInit_An_Sns : Constant  Value=0
  StePw_B_Rq : Constant  Value=0
  bus_creator : BusCreator  Inputs=6
  out_port : Outport
  wires:
  bus_creator/1 -> out_port/1  "Subsystem2"
  StePinRelInit_An_Sns/1 -> bus_creator/1  "StePinRelInit_An_Sns"
  StePw_B_Rq/1 -> bus_creator/2  "StePw_B_Rq"
  StePinComp_An_Est/1 -> bus_creator/3  "StePinComp_An_Est"
  StePinAn_No_Cs/1 -> bus_creator/4  "StePinAn_No_Cs"
  StePinAn_No_Cnt/1 -> bus_creator/5  "StePinAn_No_Cnt"
  StePinCompAnEst_D_Qf/1 -> bus_creator/6  "StePinCompAnEst_D_Qf"

== system P702_NI_SoftECU/Output/Subsystem2/CAN_Signal/PSCM/TesterPhysicalResPSCM_0x738 ==
  TesterPhysicalResPSCM : Constant  Value=0
  bus_creator : BusCreator  Inputs=1
  out_port : Outport
  wires:
  bus_creator/1 -> out_port/1  "Subsystem2"
  TesterPhysicalResPSCM/1 -> bus_creator/1  "TesterPhysicalResPSCM"

== system P702_NI_SoftECU/Output/Subsystem2/CAN_Signal/PSCM/TrailerAid_Data2_0x417 ==
  EsaOn_B_Stat : Constant  Value=0
  HitchToTrlrAxle_L_Calc : Constant  Value=0
  LatCtlLim_D_Stat : Constant  Value=0
  LatCtlSte_D_Stat : Constant  Value=0
  SelDrvMdeSte_D_Stat : Constant  Value=0
  TrlrAidEnbl_D2_Stat : Constant  Value=0
  TrlrAidMsgTxt_D2_Rq : Constant  Value=0
  TrlrAidSetup_D2_Stat : Constant  Value=0
  TrlrAidTrgtId_No_Rq : Constant  Value=0
  TrlrAidTrlrId_No_Rq : Constant  Value=0
  TrlrAnOffst_An2_Calc : Constant  Value=0
  TrlrAn_An_MxCalc : Constant  Value=0
  TrlrAn_An_WarnCalc : Constant  Value=0
  bus_creator : BusCreator  Inputs=13
  out_port : Outport
  wires:
  bus_creator/1 -> out_port/1  "Subsystem2"
  HitchToTrlrAxle_L_Calc/1 -> bus_creator/1  "HitchToTrlrAxle_L_Calc"
  TrlrAidMsgTxt_D2_Rq/1 -> bus_creator/2  "TrlrAidMsgTxt_D2_Rq"
  EsaOn_B_Stat/1 -> bus_creator/3  "EsaOn_B_Stat"
  LatCtlLim_D_Stat/1 -> bus_creator/4  "LatCtlLim_D_Stat"
  LatCtlSte_D_Stat/1 -> bus_creator/5  "LatCtlSte_D_Stat"
  SelDrvMdeSte_D_Stat/1 -> bus_creator/6  "SelDrvMdeSte_D_Stat"
  TrlrAidEnbl_D2_Stat/1 -> bus_creator/7  "TrlrAidEnbl_D2_Stat"
  TrlrAn_An_WarnCalc/1 -> bus_creator/8  "TrlrAn_An_WarnCalc"
  TrlrAnOffst_An2_Calc/1 -> bus_creator/9  "TrlrAnOffst_An2_Calc"
  TrlrAidSetup_D2_Stat/1 -> bus_creator/10  "TrlrAidSetup_D2_Stat"
  TrlrAidTrgtId_No_Rq/1 -> bus_creator/11  "TrlrAidTrgtId_No_Rq"
  TrlrAn_An_MxCalc/1 -> bus_creator/12  "TrlrAn_An_MxCalc"
  TrlrAidTrlrId_No_Rq/1 -> bus_creator/13  "TrlrAidTrlrId_No_Rq"

== system P702_NI_SoftECU/Output/Subsystem2/CAN_Signal/RealPCM/EngBrakeData ==
  CcStat_D_Actl : Constant  Value=0
  bus_creator : BusCreator  Inputs=1
  out_port : Outport
  wires:
  bus_creator/1 -> out_port/1  "Subsystem2"
  CcStat_D_Actl/1 -> bus_creator/1  "CcStat_D_Actl"

== system P702_NI_SoftECU/Output/Subsystem2/CAN_Signal/RealPCM/EngVehicleSpThrottle2 ==
  Veh_V_ActlEng : Constant  Value=0
  bus_creator : BusCreator  Inputs=1
  out_port : Outport
  wires:
  bus_creator/1 -> out_port/1  "Subsystem2"
  Veh_V_ActlEng/1 -> bus_creator/1  "Veh_V_ActlEng"

== system P702_NI_SoftECU/Output/Subsystem2/CAN_Signal/RealPCM/user_channel ==
  Desired_Speed : Constant  Value=0
  PCM_status_user_input : Constant  Value=0
  bus_creator : BusCreator  Inputs=2
  out_port : Outport
  wires:
  bus_creator/1 -> out_port/1  "Subsystem2"
  PCM_status_user_input/1 -> bus_creator/1  "PCM_status_user_input"
  Desired_Speed/1 -> bus_creator/2  "Desired_Speed"

== system P702_NI_SoftECU/Output/Subsystem2/To_NI_HIL/DSMC/DrvStatMonData ==
  DrvEngLvlConfid_D_Stat : Constant  Value=0
  DrvEngageLevel_No_Cnt : Constant  Value=0
  DrvEngageLevel_No_Cs : Constant  Value=0
  bus_creator : BusCreator  Inputs=3
  out_port : Outport
  wires:
  bus_creator/1 -> out_port/1  "Subsystem2"
  DrvEngLvlConfid_D_Stat/1 -> bus_creator/1  "DrvEngLvlConfid_D_Stat"
  DrvEngageLevel_No_Cs/1 -> bus_creator/2  "DrvEngageLevel_No_Cs"
  DrvEngageLevel_No_Cnt/1 -> bus_creator/3  "DrvEngageLevel_No_Cnt"

== system P702_NI_SoftECU/Output/Subsystem2/To_NI_HIL/SRR_L/FL_SOD ==
  SRR_FL_001 : Subsystem
  SRR_FL_002 : Subsystem
  SRR_FL_003 : Subsystem
  bus_creator : BusCreator  Inputs=3
  out_port : Outport
  wires:
  bus_creator/1 -> out_port/1  "Subsystem2"
  SRR_FL_001/1(out_port) -> bus_creator/1  "SRR_FL_001"
  SRR_FL_002/1(out_port) -> bus_creator/2  "SRR_FL_002"
  SRR_FL_003/1(out_port) -> bus_creator/3  "SRR_FL_003"

== system P702_NI_SoftECU/Output/Subsystem2/To_NI_HIL/SRR_L/RL_SOD ==
  SRR_RL_001 : Subsystem
  SRR_RL_002 : Subsystem
  SRR_RL_003 : Subsystem
  bus_creator : BusCreator  Inputs=3
  out_port : Outport
  wires:
  bus_creator/1 -> out_port/1  "Subsystem2"
  SRR_RL_001/1(out_port) -> bus_creator/1  "SRR_RL_001"
  SRR_RL_002/1(out_port) -> bus_creator/2  "SRR_RL_002"
  SRR_RL_003/1(out_port) -> bus_creator/3  "SRR_RL_003"

== system P702_NI_SoftECU/Output/Subsystem2/To_NI_HIL/SRR_R/FR_SOD ==
  SRR_FR_001 : Subsystem
  SRR_FR_002 : Subsystem
  SRR_FR_003 : Subsystem
  bus_creator : BusCreator  Inputs=3
  out_port : Outport
  wires:
  bus_creator/1 -> out_port/1  "Subsystem2"
  SRR_FR_001/1(out_port) -> bus_creator/1  "SRR_FR_001"
  SRR_FR_002/1(out_port) -> bus_creator/2  "SRR_FR_002"
  SRR_FR_003/1(out_port) -> bus_creator/3  "SRR_FR_003"

== system P702_NI_SoftECU/Output/Subsystem2/To_NI_HIL/SRR_R/RR_SOD ==
  SRR_RR_001 : Subsystem
  SRR_RR_002 : Subsystem
  SRR_RR_003 : Subsystem
  bus_creator : BusCreator  Inputs=3
  out_port : Outport
  wires:
  bus_creator/1 -> out_port/1  "Subsystem2"
  SRR_RR_001/1(out_port) -> bus_creator/1  "SRR_RR_001"
  SRR_RR_002/1(out_port) -> bus_creator/2  "SRR_RR_002"
  SRR_RR_003/1(out_port) -> bus_creator/3  "SRR_RR_003"

== system P702_NI_SoftECU/Output/Subsystem2/To_NI_HIL/Soft_ABS/ABS_BrkBst_Data ==
  BrkTotTqRqDrv_No_Cnt : Constant  Value=0
  BrkTotTqRqDrv_No_Cs : Constant  Value=0
  BrkTot_Tq_RqDrv : Constant  Value=0
  bus_creator : BusCreator  Inputs=3
  out_port : Outport
  wires:
  bus_creator/1 -> out_port/1  "Subsystem2"
  BrkTot_Tq_RqDrv/1 -> bus_creator/1  "BrkTot_Tq_RqDrv"
  BrkTotTqRqDrv_No_Cs/1 -> bus_creator/2  "BrkTotTqRqDrv_No_Cs"
  BrkTotTqRqDrv_No_Cnt/1 -> bus_creator/3  "BrkTotTqRqDrv_No_Cnt"

== system P702_NI_SoftECU/Output/Subsystem2/To_NI_HIL/Soft_ABS/Accel_Data ==
  VehLat2_A_Actl : Constant  Value=0
  VehLong2_A_Actl : Constant  Value=0
  bus_creator : BusCreator  Inputs=2
  out_port : Outport
  wires:
  bus_creator/1 -> out_port/1  "Subsystem2"
  VehLong2_A_Actl/1 -> bus_creator/1  "VehLong2_A_Actl"
  VehLat2_A_Actl/1 -> bus_creator/2  "VehLat2_A_Actl"

== system P702_NI_SoftECU/Output/Subsystem2/To_NI_HIL/Soft_ABS/BrakeSnData_3 ==
  VehLatComp_A_Actl : Constant  Value=0
  VehLongComp_A_Actl : Constant  Value=0
  VehOverGnd_V_Est : Constant  Value=0
  VehYawComp_W_Actl : Constant  Value=0
  bus_creator : BusCreator  Inputs=4
  out_port : Outport
  wires:
  bus_creator/1 -> out_port/1  "Subsystem2"
  VehYawComp_W_Actl/1 -> bus_creator/1  "VehYawComp_W_Actl"
  VehOverGnd_V_Est/1 -> bus_creator/2  "VehOverGnd_V_Est"
  VehLongComp_A_Actl/1 -> bus_creator/3  "VehLongComp_A_Actl"
  VehLatComp_A_Actl/1 -> bus_creator/4  "VehLatComp_A_Actl"

== system P702_NI_SoftECU/Output/Subsystem2/To_NI_HIL/Soft_ABS/BrakeSnData_4 ==
  BrkTot_Tq_Actl : Constant  Value=0
  VehRolComp_W_Actl : Constant  Value=0
  VehVertComp_A_Actl : Constant  Value=0
  bus_creator : BusCreator  Inputs=3
  out_port : Outport
  wires:
  bus_creator/1 -> out_port/1  "Subsystem2"
  VehVertComp_A_Actl/1 -> bus_creator/1  "VehVertComp_A_Actl"
  VehRolComp_W_Actl/1 -> bus_creator/2  "VehRolComp_W_Actl"
  BrkTot_Tq_Actl/1 -> bus_creator/3  "BrkTot_Tq_Actl"

== system P702_NI_SoftECU/Output/Subsystem2/To_NI_HIL/Soft_ABS/BrakeSnData_5 ==
  SteWhlComp_An_Est : Constant  Value=0
  bus_creator : BusCreator  Inputs=1
  out_port : Outport
  wires:
  bus_creator/1 -> out_port/1  "Subsystem2"
  SteWhlComp_An_Est/1 -> bus_creator/1  "SteWhlComp_An_Est"

== system P702_NI_SoftECU/Output/Subsystem2/To_NI_HIL/Soft_ABS/BrakeSysFeatures ==
  VehVActlBrk_No_Cnt : Constant  Value=0
  VehVActlBrk_No_Cs : Constant  Value=0
  Veh_V_ActlBrk : Constant  Value=0
  bus_creator : BusCreator  Inputs=3
  out_port : Outport
  wires:
  bus_creator/1 -> out_port/1  "Subsystem2"
  Veh_V_ActlBrk/1 -> bus_creator/1  "Veh_V_ActlBrk"
  VehVActlBrk_No_Cs/1 -> bus_creator/2  "VehVActlBrk_No_Cs"
  VehVActlBrk_No_Cnt/1 -> bus_creator/3  "VehVActlBrk_No_Cnt"

== system P702_NI_SoftECU/Output/Subsystem2/To_NI_HIL/Soft_ABS/BrakeSysFeatures_2 ==
  BpedMove_D_Actl : Constant  Value=0
  BpedMove_No_Cnt : Constant  Value=0
  BpedMove_No_Cs : Constant  Value=0
  bus_creator : BusCreator  Inputs=3
  out_port : Outport
  wires:
  bus_creator/1 -> out_port/1  "Subsystem2"
  BpedMove_D_Actl/1 -> bus_creator/1  "BpedMove_D_Actl"
  BpedMove_No_Cs/1 -> bus_creator/2  "BpedMove_No_Cs"
  BpedMove_No_Cnt/1 -> bus_creator/3  "BpedMove_No_Cnt"

== system P702_NI_SoftECU/Output/Subsystem2/To_NI_HIL/Soft_ABS/DesiredTorqBrk ==
  AccBrkActv_B_Actl : Constant  Value=0
  AccBrkPrchgActv_B_Actl : Constant  Value=0
  AccBrkTotTqMn_B_Actl : Constant  Value=0
  AccStopActv_B_ActlBrk : Constant  Value=0
  CmbbBaSensInc_B_Actl : Constant  Value=0
  CmbbBrkDecel_B_Actl : Constant  Value=0
  CmbbBrkPrchg_B_Actl : Constant  Value=0
  VehLongOvrGnd_A_Est : Constant  Value=0
  VehStop_D_Stat : Constant  Value=0
  VehicleStationary : Constant  Value=0
  bus_creator : BusCreator  Inputs=10
  out_port : Outport
  wires:
  bus_creator/1 -> out_port/1  "Subsystem2"
  AccBrkPrchgActv_B_Actl/1 -> bus_creator/1  "AccBrkPrchgActv_B_Actl"
  AccBrkActv_B_Actl/1 -> bus_creator/2  "AccBrkActv_B_Actl"
  AccStopActv_B_ActlBrk/1 -> bus_creator/3  "AccStopActv_B_ActlBrk"
  CmbbBrkPrchg_B_Actl/1 -> bus_creator/4  "CmbbBrkPrchg_B_Actl"
  CmbbBaSensInc_B_Actl/1 -> bus_creator/5  "CmbbBaSensInc_B_Actl"
  CmbbBrkDecel_B_Actl/1 -> bus_creator/6  "CmbbBrkDecel_B_Actl"
  VehicleStationary/1 -> bus_creator/7  "VehicleStationary"
  VehStop_D_Stat/1 -> bus_creator/8  "VehStop_D_Stat"
  VehLongOvrGnd_A_Est/1 -> bus_creator/9  "VehLongOvrGnd_A_Est"
  AccBrkTotTqMn_B_Actl/1 -> bus_creator/10  "AccBrkTotTqMn_B_Actl"

== system P702_NI_SoftECU/Output/Subsystem2/To_NI_HIL/Soft_ABS/ToCarSim ==
  MCPressure : Constant  Value=0
  bus_creator : BusCreator  Inputs=1
  out_port : Outport
  wires:
  bus_creator/1 -> out_port/1  "Subsystem2"
  MCPressure/1 -> bus_creator/1  "MCPressure"

== system P702_NI_SoftECU/Output/Subsystem2/To_NI_HIL/Soft_ABS/WheelData ==
  WhlDirRl_D_Actl : Constant  Value=0
  WhlDirRr_D_Actl : Constant  Value=0
  bus_creator : BusCreator  Inputs=2
  out_port : Outport
  wires:
  bus_creator/1 -> out_port/1  "Subsystem2"
  WhlDirRl_D_Actl/1 -> bus_creator/1  "WhlDirRl_D_Actl"
  WhlDirRr_D_Actl/1 -> bus_creator/2  "WhlDirRr_D_Actl"

== system P702_NI_SoftECU/Output/Subsystem2/To_NI_HIL/Soft_ABS/WheelSpeed ==
  WhlFl_W_Meas : Constant  Value=0
  WhlFr_W_Meas : Constant  Value=0
  WhlRl_W_Meas : Constant  Value=0
  WhlRotatFl_No_Cnt : Constant  Value=0
  WhlRotatFr_No_Cnt : Constant  Value=0
  WhlRotatRl_No_Cnt : Constant  Value=0
  WhlRotatRr_No_Cnt : Constant  Value=0
  WhlRr_W_Meas : Constant  Value=0
  bus_creator : BusCreator  Inputs=8
  out_port : Outport
  wires:
  bus_creator/1 -> out_port/1  "Subsystem2"
  WhlFl_W_Meas/1 -> bus_creator/1  "WhlFl_W_Meas"
  WhlFr_W_Meas/1 -> bus_creator/2  "WhlFr_W_Meas"
  WhlRl_W_Meas/1 -> bus_creator/3  "WhlRl_W_Meas"
  WhlRr_W_Meas/1 -> bus_creator/4  "WhlRr_W_Meas"
  WhlRotatFl_No_Cnt/1 -> bus_creator/5  "WhlRotatFl_No_Cnt"
  WhlRotatFr_No_Cnt/1 -> bus_creator/6  "WhlRotatFr_No_Cnt"
  WhlRotatRl_No_Cnt/1 -> bus_creator/7  "WhlRotatRl_No_Cnt"
  WhlRotatRr_No_Cnt/1 -> bus_creator/8  "WhlRotatRr_No_Cnt"

== system P702_NI_SoftECU/Output/Subsystem2/To_NI_HIL/Soft_ABS/Yaw_Data ==
  VehYaw_W_Actl : Constant  Value=0
  bus_creator : BusCreator  Inputs=1
  out_port : Outport
  wires:
  bus_creator/1 -> out_port/1  "Subsystem2"
  VehYaw_W_Actl/1 -> bus_creator/1  "VehYaw_W_Actl"

== system P702_NI_SoftECU/Output/Subsystem2/To_NI_HIL/Soft_BCM/BodyInfo_3 ==
  Ignition_Status : Constant  Value=0
  bus_creator : BusCreator  Inputs=1
  out_port : Outport
  wires:
  bus_creator/1 -> out_port/1  "Subsystem2"
  Ignition_Status/1 -> bus_creator/1  "Ignition_Status"

== system P702_NI_SoftECU/Output/Subsystem2/To_NI_HIL/Soft_BCM/Cluster_Info1 ==
  OdometerMasterValue : Constant  Value=0
  OdometerMasterValue_UB : Constant  Value=0
  bus_creator : BusCreator  Inputs=2
  out_port : Outport
  wires:
  bus_creator/1 -> out_port/1  "Subsystem2"
  OdometerMasterValue/1 -> bus_creator/1  "OdometerMasterValue"
  OdometerMasterValue_UB/1 -> bus_creator/2  "OdometerMasterValue_UB"

== system P702_NI_SoftECU/Output/Subsystem2/To_NI_HIL/Soft_BCM/GGCC_Config_Mgmt_ID ==
  Byte_{0..7} (8 alike) : Constant  Value=0
  bus_creator : BusCreator  Inputs=8
  out_port : Outport
  wires:
  bus_creator/1 -> out_port/1  "Subsystem2"
  Byte_0/1 -> bus_creator/1  "Byte_0"
  Byte_1/1 -> bus_creator/2  "Byte_1"
  Byte_2/1 -> bus_creator/3  "Byte_2"
  Byte_3/1 -> bus_creator/4  "Byte_3"
  Byte_4/1 -> bus_creator/5  "Byte_4"
  Byte_5/1 -> bus_creator/6  "Byte_5"
  Byte_6/1 -> bus_creator/7  "Byte_6"
  Byte_7/1 -> bus_creator/8  "Byte_7"

== system P702_NI_SoftECU/Output/Subsystem2/To_NI_HIL/Soft_BCM/Personality_BCM2_Data ==
  RecallEvent_No_Cnt : Constant  Value=0
  bus_creator : BusCreator  Inputs=1
  out_port : Outport
  wires:
  bus_creator/1 -> out_port/1  "Subsystem2"
  RecallEvent_No_Cnt/1 -> bus_creator/1  "RecallEvent_No_Cnt"

== system P702_NI_SoftECU/Output/Subsystem2/To_NI_HIL/Soft_ECM/EngBrakeData ==
  ACCStopMde_D_Rq : Constant  Value=0
  Cc_Stat_D_Actl : Constant  Value=0
  CmbbEngTqMn_B_Rq : Constant  Value=0
  PrplTqMnSat_B_Actl : Constant  Value=0
  bus_creator : BusCreator  Inputs=4
  out_port : Outport
  wires:
  bus_creator/1 -> out_port/1  "Subsystem2"
  CmbbEngTqMn_B_Rq/1 -> bus_creator/1  "CmbbEngTqMn_B_Rq"
  ACCStopMde_D_Rq/1 -> bus_creator/2  "ACCStopMde_D_Rq"
  PrplTqMnSat_B_Actl/1 -> bus_creator/3  "PrplTqMnSat_B_Actl"
  Cc_Stat_D_Actl/1 -> bus_creator/4  "Cc_Stat_D_Actl"

== system P702_NI_SoftECU/Output/Subsystem2/To_NI_HIL/Soft_ECM/EngVehicleSpThrottle ==
  EngAout_N_Actl : Constant  Value=0
  bus_creator : BusCreator  Inputs=1
  out_port : Outport
  wires:
  bus_creator/1 -> out_port/1  "Subsystem2"
  EngAout_N_Actl/1 -> bus_creator/1  "EngAout_N_Actl"

== system P702_NI_SoftECU/Output/Subsystem2/To_NI_HIL/Soft_ECM/EngVehicleSpThrottle2 ==
  Veh_V_ActlEng : Constant  Value=0
  bus_creator : BusCreator  Inputs=1
  out_port : Outport
  wires:
  bus_creator/1 -> out_port/1  "Subsystem2"
  Veh_V_ActlEng/1 -> bus_creator/1  "Veh_V_ActlEng"

== system P702_NI_SoftECU/Output/Subsystem2/To_NI_HIL/Soft_MRR/MRR_Detection ==
  MRR_Detection_001 : Subsystem
  MRR_Detection_002 : Subsystem
  MRR_Detection_003 : Subsystem
  bus_creator : BusCreator  Inputs=3
  out_port : Outport
  wires:
  bus_creator/1 -> out_port/1  "Subsystem2"
  MRR_Detection_001/1(out_port) -> bus_creator/1  "MRR_Detection_001"
  MRR_Detection_002/1(out_port) -> bus_creator/2  "MRR_Detection_002"
  MRR_Detection_003/1(out_port) -> bus_creator/3  "MRR_Detection_003"

== system P702_NI_SoftECU/Output/Subsystem2/To_NI_HIL/Soft_PCM/EngBrakeData ==
  BpedDrvAppl_D_Actl : Constant  Value=0
  BrkOnOffSwtch_D_Actl : Constant  Value=0
  bus_creator : BusCreator  Inputs=2
  out_port : Outport
  wires:
  bus_creator/1 -> out_port/1  "Subsystem2"
  BrkOnOffSwtch_D_Actl/1 -> bus_creator/1  "BrkOnOffSwtch_D_Actl"
  BpedDrvAppl_D_Actl/1 -> bus_creator/2  "BpedDrvAppl_D_Actl"

== system P702_NI_SoftECU/Output/Subsystem2/To_NI_HIL/Soft_PCM/EngVehicleSpThottle2 ==
  GearRvrse_D_Actl : Constant  Value=0
  Veh_V_ActlEng : Constant  Value=0
  Veh_V_RqCcSet : Constant  Value=0
  bus_creator : BusCreator  Inputs=3
  out_port : Outport
  wires:
  bus_creator/1 -> out_port/1  "Subsystem2"
  Veh_V_ActlEng/1 -> bus_creator/1  "Veh_V_ActlEng"
  GearRvrse_D_Actl/1 -> bus_creator/2  "GearRvrse_D_Actl"
  Veh_V_RqCcSet/1 -> bus_creator/3  "Veh_V_RqCcSet"

== system P702_NI_SoftECU/Output/Subsystem2/To_NI_HIL/Soft_PCM/EngVehicleSpThrottle ==
  ApedPosPcActl_No_Cs : Constant  Value=0
  ApedPos_PcRate_ActlArb : Constant  Value=0
  ApedPos_Pc_ActlArb : Constant  Value=0
  ApedPos_Pc_ActlArb_No_Cnt : Constant  Value=0
  EngAout_N_Actl : Constant  Value=0
  bus_creator : BusCreator  Inputs=5
  out_port : Outport
  wires:
  bus_creator/1 -> out_port/1  "Subsystem2"
  EngAout_N_Actl/1 -> bus_creator/1  "EngAout_N_Actl"
  ApedPos_Pc_ActlArb/1 -> bus_creator/2  "ApedPos_Pc_ActlArb"
  ApedPos_PcRate_ActlArb/1 -> bus_creator/3  "ApedPos_PcRate_ActlArb"
  ApedPosPcActl_No_Cs/1 -> bus_creator/4  "ApedPosPcActl_No_Cs"
  ApedPos_Pc_ActlArb_No_Cnt/1 -> bus_creator/5  "ApedPos_Pc_ActlArb_No_Cnt"

== system P702_NI_SoftECU/Output/Subsystem2/To_NI_HIL/Soft_PCM/EngineClimateData ==
  AirAmb_Te_Actl : Constant  Value=0
  AirAmb_Te_ActlFilt : Constant  Value=0
  EngAout_Aa_Actl : Constant  Value=0
  bus_creator : BusCreator  Inputs=3
  out_port : Outport
  wires:
  bus_creator/1 -> out_port/1  "Subsystem2"
  EngAout_Aa_Actl/1 -> bus_creator/1  "EngAout_Aa_Actl"
  AirAmb_Te_Actl/1 -> bus_creator/2  "AirAmb_Te_Actl"
  AirAmb_Te_ActlFilt/1 -> bus_creator/3  "AirAmb_Te_ActlFilt"

== system P702_NI_SoftECU/Output/Subsystem2/To_NI_HIL/Soft_PCM/EngineClutchData ==
  CluPdlPosPcMeas_D_Qf : Constant  Value=0
  CluPdlPos_Pc_Meas : Constant  Value=0
  CluPdl_PcRate_Actl : Constant  Value=0
  bus_creator : BusCreator  Inputs=3
  out_port : Outport
  wires:
  bus_creator/1 -> out_port/1  "Subsystem2"
  CluPdl_PcRate_Actl/1 -> bus_creator/1  "CluPdl_PcRate_Actl"
  CluPdlPos_Pc_Meas/1 -> bus_creator/2  "CluPdlPos_Pc_Meas"
  CluPdlPosPcMeas_D_Qf/1 -> bus_creator/3  "CluPdlPosPcMeas_D_Qf"

== system P702_NI_SoftECU/Output/Subsystem2/To_NI_HIL/Soft_PCM/EngineData_7 ==
  FuelFlw_Vl_Dsply : Constant  Value=0
  OdoCount : Constant  Value=0
  bus_creator : BusCreator  Inputs=2
  out_port : Outport
  wires:
  bus_creator/1 -> out_port/1  "Subsystem2"
  OdoCount/1 -> bus_creator/1  "OdoCount"
  FuelFlw_Vl_Dsply/1 -> bus_creator/2  "FuelFlw_Vl_Dsply"

== system P702_NI_SoftECU/Output/Subsystem2/To_NI_HIL/Soft_PCM/PowertrainData_10 ==
  GearLvr_D_ActlDrv : Constant  Value=0
  GearPos_No_Cnt : Constant  Value=0
  GearPos_No_Cs : Constant  Value=0
  bus_creator : BusCreator  Inputs=3
  out_port : Outport
  wires:
  bus_creator/1 -> out_port/1  "Subsystem2"
  GearPos_No_Cs/1 -> bus_creator/1  "GearPos_No_Cs"
  GearPos_No_Cnt/1 -> bus_creator/2  "GearPos_No_Cnt"
  GearLvr_D_ActlDrv/1 -> bus_creator/3  "GearLvr_D_ActlDrv"

== system P702_NI_SoftECU/Output/Subsystem2/To_NI_HIL/Soft_PCM/TorqueDataEngFlags ==
  PrplWhlTotTqRq_No_Cs : Constant  Value=0
  PrplWhlTot_Tq_Rq : Constant  Value=0
  PrplWhlTot_Tq_Rq_No_Cnt : Constant  Value=0
  bus_creator : BusCreator  Inputs=3
  out_port : Outport
  wires:
  bus_creator/1 -> out_port/1  "Subsystem2"
  PrplWhlTot_Tq_Rq/1 -> bus_creator/1  "PrplWhlTot_Tq_Rq"
  PrplWhlTotTqRq_No_Cs/1 -> bus_creator/2  "PrplWhlTotTqRq_No_Cs"
  PrplWhlTot_Tq_Rq_No_Cnt/1 -> bus_creator/3  "PrplWhlTot_Tq_Rq_No_Cnt"

== system P702_NI_SoftECU/Output/Subsystem2/To_NI_HIL/Soft_PCM/VehicleOperatingModes ==
  ElPw_D_Stat : Constant  Value=0
  ElPw_D_StatStrtStop : Constant  Value=0
  Eng_D_Stat : Constant  Value=0
  PrplWhlTot2_Tq_Rq : Constant  Value=0
  PwPckTq_D_Stat : Constant  Value=0
  bus_creator : BusCreator  Inputs=5
  out_port : Outport
  wires:
  bus_creator/1 -> out_port/1  "Subsystem2"
  Eng_D_Stat/1 -> bus_creator/1  "Eng_D_Stat"
  PwPckTq_D_Stat/1 -> bus_creator/2  "PwPckTq_D_Stat"
  PrplWhlTot2_Tq_Rq/1 -> bus_creator/3  "PrplWhlTot2_Tq_Rq"
  ElPw_D_StatStrtStop/1 -> bus_creator/4  "ElPw_D_StatStrtStop"
  ElPw_D_Stat/1 -> bus_creator/5  "ElPw_D_Stat"

== system P702_NI_SoftECU/Output/Subsystem2/To_NI_HIL/Soft_RCM/Accel_Data ==
  VehLat2_A_Actl : Constant  Value=0
  VehLatAActl_D_Qf : Constant  Value=0
  VehLatLongVert_No_Cnt : Constant  Value=0
  VehLatLongVert_No_Cs : Constant  Value=0
  VehLong2_A_Actl : Constant  Value=0
  VehLongAActl_D_Qf : Constant  Value=0
  VehVert2_A_Actl : Constant  Value=0
  VehVertAActl_D_Qf : Constant  Value=0
  bus_creator : BusCreator  Inputs=8
  out_port : Outport
  wires:
  bus_creator/1 -> out_port/1  "Subsystem2"
  VehLat2_A_Actl/1 -> bus_creator/1  "VehLat2_A_Actl"
  VehLong2_A_Actl/1 -> bus_creator/2  "VehLong2_A_Actl"
  VehVert2_A_Actl/1 -> bus_creator/3  "VehVert2_A_Actl"
  VehLatLongVert_No_Cnt/1 -> bus_creator/4  "VehLatLongVert_No_Cnt"
  VehLatLongVert_No_Cs/1 -> bus_creator/5  "VehLatLongVert_No_Cs"
  VehLatAActl_D_Qf/1 -> bus_creator/6  "VehLatAActl_D_Qf"
  VehLongAActl_D_Qf/1 -> bus_creator/7  "VehLongAActl_D_Qf"
  VehVertAActl_D_Qf/1 -> bus_creator/8  "VehVertAActl_D_Qf"

== system P702_NI_SoftECU/Output/Subsystem2/To_NI_HIL/Soft_RCM/RCMStatusMessage2 ==
  FirstRowBuckleDriver : Constant  Value=0
  RstrnImpactEvntStatus : Constant  Value=0
  bus_creator : BusCreator  Inputs=2
  out_port : Outport
  wires:
  bus_creator/1 -> out_port/1  "Subsystem2"
  RstrnImpactEvntStatus/1 -> bus_creator/1  "RstrnImpactEvntStatus"
  FirstRowBuckleDriver/1 -> bus_creator/2  "FirstRowBuckleDriver"

== system P702_NI_SoftECU/Output/Subsystem2/To_NI_HIL/Soft_RCM/Yaw_Data ==
  VehRolWActl_D_Qf : Constant  Value=0
  VehRol_W_Actl : Constant  Value=0
  VehRollYawW_No_Cs : Constant  Value=0
  VehRollYaw_No_Cnt : Constant  Value=0
  VehYawWActl_D_Qf : Constant  Value=0
  VehYaw_W_Actl : Constant  Value=0
  bus_creator : BusCreator  Inputs=6
  out_port : Outport
  wires:
  bus_creator/1 -> out_port/1  "Subsystem2"
  VehRol_W_Actl/1 -> bus_creator/1  "VehRol_W_Actl"
  VehYaw_W_Actl/1 -> bus_creator/2  "VehYaw_W_Actl"
  VehRollYaw_No_Cnt/1 -> bus_creator/3  "VehRollYaw_No_Cnt"
  VehRollYawW_No_Cs/1 -> bus_creator/4  "VehRollYawW_No_Cs"
  VehRolWActl_D_Qf/1 -> bus_creator/5  "VehRolWActl_D_Qf"
  VehYawWActl_D_Qf/1 -> bus_creator/6  "VehYawWActl_D_Qf"
